simulink model "PMSM_Ld"  (R2024a)
settings: Solver=FixedStepAuto  StartTime=0.0  StopTime=0.5  FixedStep=1E-6  RelTol=1e-3
model workspace (MAT data in the model file):
  PWM_Frequency = Simulink.Parameter
  PWM_Frequency.Value = 30000
  PWM_Frequency.Complexity = 'real'
  PWM_Frequency.Dimensions = [1 1]
  PWM_Frequency.DataType = 'double'
  TimerPeriod = 0.1
values from neighbouring files (symbols this model uses):
  Flux = 0.01837    [Flux_Nonsensor_data_new.m]
undefined symbols (not defined in the file or in its folder): Down, Up
libraries: eePwmGenerator x4, spsDCVoltageSourceLib x1, spsPermanentMagnetSynchronousMachineLib x1, spsUniversalBridgeLib x1, sps_lib x1, eeGeneralControl x1
settings Model: Creator=shish  LastModifiedBy=shish

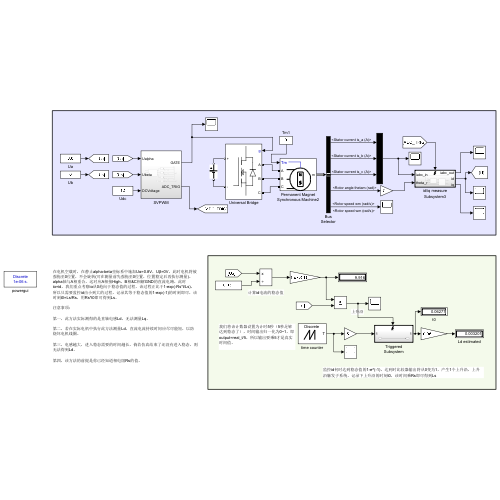
[thumbnail: Simulink's stored preview of the top-level diagram]
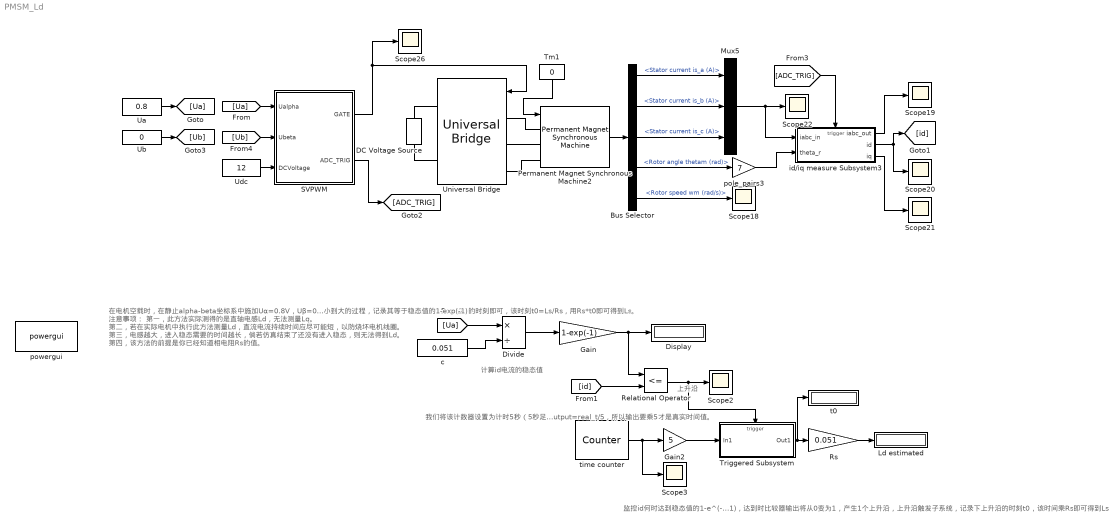
== system PMSM_Ld ==
  note: 我们将该计数器设置为计时5秒（5秒足够达到稳态了），时间输出归一化为0~1，即output=real_t/5，所以输出要乘5才是真实时间值。
  note: 上升沿
  note: 监控id何时达到稳态值的1-e^(-1)，达到时比较器输出将从0变为1，产生1个上升沿，上升沿触发子系统，记录下上升沿的时刻t0，该时间乘Rs即可得到Ls
  note: 计算id电流的稳态值
  note: 在电机空载时，在静止alpha-beta坐标系中施加Uα=0.8V，Uβ=0V，此时电机将被强拖至0位置，不会旋转(可在测量前先强拖至0位置，位置稳定后再执行测量)。alpha轴与A相重合，这对应A相接High，B相&C相解GND的直流电路，此时iα=id，我们重点考察iα从0趋向于稳态值的过程，该过程正比于1-exp(-Rs*t/Ls)，所以只需要监控id由小到大的过程，记录其等于稳态值的1-exp(-1)的时刻即可，该时刻t0=Ls/Rs，用Rs*t0即可得到Ls。
      |
      | 注意事项：
      |
      | 第一，此方法实际测得的是直轴电感Ld，无法测量Lq。
      |
      | 第二，若在实际电机中执行此方法测量Ld，直流电流持续时间应尽可能短，以防烧坏电机线圈。
      |
      | 第三，电感越大，进入稳态需要的时间越长，倘若仿真结束了还没有进入稳态，则无法得到Ld。
      |
      | 第四，该方法的前提是你已经知道相电阻Rs的值。
  " c" : Constant  Value=0.051
  Bus Selector : BusSelector  OutputSignals=Stator current is_a (A),Stator current is_b (A),Stator current is_c (A),Rotor angle thetam (rad),Rotor speed wm (rad/s)
  DC Voltage Source : spsDCVoltageSourceLib/DC Voltage Source  Amplitude=12  Measurements=Voltage
  Display : Display
  Divide : Product  Inputs=*/
  Gain : Gain  Gain=1-exp(-1)
  Gain2 : Gain  Gain=5
  Ld estimated : Display
  Mux5 : Mux  Inputs=3
  Permanent Magnet Synchronous Machine2 : spsPermanentMagnetSynchronousMachineLib/Permanent Magnet Synchronous Machine  NbPhases=3  FluxDistribution=Sinusoidal  RotorType=Salient-pole  MechanicalLoad=Torque Tm  PresetModel=No  ShowDetailedParameters=on  MeasurementBus=off  Resistance=0.05  Inductance=8.5e-3  dqInductances=[3.2e-3,1.8e-3]  La=0.000395  MachineConstant=Flux linkage established by magnets (V.s)  Flux=0.00012  VoltageCst=0.15236  TorqueCst=0.00126  Flat=120  Mechanical=[0.000012 0.000005 7 0]  PolePairs=4  InitialConditions=[0,0,0,0]  InitialConditions5ph=[0 0 0 0 0 0]  RefAngle=Aligned with phase A axis (original Park)  IterativeDiscreteModel=Trapezoidal non iterative  TsBlock=-1  TsPowergui=0
  Relational Operator : RelationalOperator  Operator=<=  OutDataTypeStr=boolean  RndMeth=Simplest  InputSameDT=off
  Rs : Gain  Gain=0.051
  SVPWM : Subsystem
  Scope{2..3,18..22,26} (8 alike) : Scope
  Tm1 : Constant  Value=0
  Triggered Subsystem : Subsystem  TreatAsAtomicUnit=on
  Ua : Constant  Value=0.8
  Ub : Constant  Value=0
  Udc : Constant  Value=12
  Universal Bridge : spsUniversalBridgeLib/Universal Bridge  Arms=3  SnubberResistance=1e5  SnubberCapacitance=inf  Device=MOSFET / Diodes  Ron=1e-3  Lon=0  ForwardVoltages="[  0  0  ]"  ForwardVoltage=0  GTOparameters=[ 10e-6 , 20e-6 ]  IGBTparameters=[ 1e-6 , 2e-6 ]  Measurements=None  Measurements_2=None  converterType=Rectifier
  id/iq measure Subsystem3 : Subsystem  TreatAsAtomicUnit=on
  pole_pairs3 : Gain  Gain=7
  powergui : sps_lib/powergui  Priority=1  SimulationMode=Discrete  SampleTime=1e-6  frequency=60  Iterations=50  frequencyindice=0  Pbase=100e6  ErrMax=1e-4  UnitsV=kV  UnitsW=MW  buscounter=0  FunctionMessages=off  echomessages=off  EnableUseOfTLC=off  CurrentSourceSwitches=off  DisableSnubberDevices=off  DisableRonSwitches=off  DisableVfSwitches=off  DisplayEquations=off  AutomaticDiscreteSolvers=off  SolverType=Tustin/Backward Euler (TBE)  Interpol=off  ExternalGateDelay=off  methode=off  Ts=100  x0status=blocks  SPID=on  SwTol=0  HookPort=off  NonlinearTolerance=1e-4  nMaxIteration=100  ContinueOnMaxIteration=off  RestoreLinks=warning  ResistiveCurrentMeasurement=off  Frange=[0:2:500]  Ylog=off  Xlog=on  ShowGrid=off  save=off  variable=ZData  structure=0  ZoomFFT=off  StartTime=0.0  cycles=1  DisplayStyle=1  fundamental=60  FreqAxis=off  MaxFrequency=1000  frequencyindicesteady=1  RmsSteady=1  display=off
  t0 : Display
  time counter : eeGeneralControl/Counter  CarrCount=Up  Range=[0 1]  Tper=5  Tdelay=0  Ts=0.000001
      settings: LibrarySourceBlock=ee_sl_lib/General Control/Counter
  wires:
  Bus Selector/5 -> Scope18/1  "<Rotor speed wm (rad/s)>"
  Bus Selector/3 -> Mux5/3  "<Stator current is_c (A)>"
  Permanent Magnet Synchronous Machine2/1 -> Bus Selector/1
  Bus Selector/4 -> pole_pairs3/1  "<Rotor angle thetam (rad)>"
  Udc/1 -> SVPWM/3(DCVoltage)
  id/iq measure Subsystem3/1(iabc_out) -> Scope19/1
  Bus Selector/2 -> Mux5/2  "<Stator current is_b (A)>"
  Mux5/1 -> Scope22/1, id/iq measure Subsystem3/1(iabc_in)
  SVPWM/1(GATE) -> Universal Bridge/1, Scope26/1
  Bus Selector/1 -> Mux5/1  "<Stator current is_a (A)>"
  pole_pairs3/1 -> id/iq measure Subsystem3/2(theta_r)
  id/iq measure Subsystem3/2(id) -> [id], Scope20/1
  id/iq measure Subsystem3/3(iq) -> Scope21/1
  [Ua] -> SVPWM/1(Ualpha)
  [Ua] -> Divide/1
  " c"/1 -> Divide/2
  Divide/1 -> Gain/1
  Gain/1 -> Relational Operator/1, Display/1
  SVPWM/2(ADC_TRIG) -> [ADC_TRIG]
  [ADC_TRIG] -> id/iq measure Subsystem3/Trigger
  [id] -> Relational Operator/2
  Relational Operator/1 -> Triggered Subsystem/Trigger, Scope2/1
  time counter/1 -> Gain2/1, Scope3/1
  Triggered Subsystem/1(Out1) -> t0/1, Rs/1
  Rs/1 -> Ld estimated/1
  Ua/1 -> [Ua]
  Gain2/1 -> Triggered Subsystem/1(In1)
  [Ub] -> SVPWM/2(Ubeta)
  Ub/1 -> [Ub]
  Tm1/1 -> Permanent Magnet Synchronous Machine2/1
  connections:
  Universal Bridge/LConn2 -- Permanent Magnet Synchronous Machine2/LConn2
  Universal Bridge/LConn1 -- Permanent Magnet Synchronous Machine2/LConn1
  Universal Bridge/LConn3 -- Permanent Magnet Synchronous Machine2/LConn3
  DC Voltage Source/LConn1 -- Universal Bridge/RConn2
  DC Voltage Source/RConn1 -- Universal Bridge/RConn1

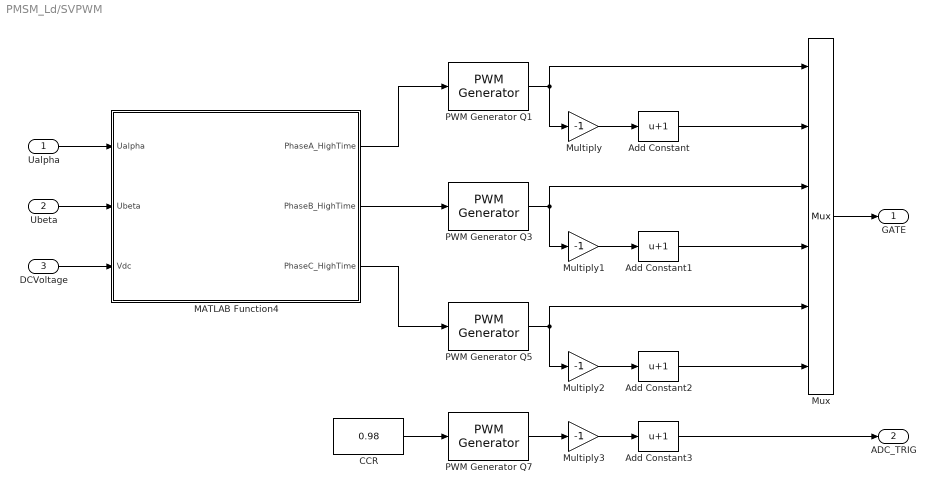
== system PMSM_Ld/SVPWM ==
  Ualpha : Inport
  Ubeta : Inport  Port=2
  DCVoltage : Inport  Port=3
  Add Constant{,1..3} (4 alike) : Bias  Bias=1  SaturateOnIntegerOverflow=off
  CCR : Constant  Value=0.98
  MATLAB Function4 : MATLAB Function  TreatAsAtomicUnit=on
  Multiply{,1..3} (4 alike) : Gain  Gain=-1
  Mux : Mux  Inputs=6
  PWM Generator Q{1,3,5,7} (4 alike) : eePwmGenerator/PWM Generator  CarrCount=Up-Down  Tper=1.0/PWM_Frequency  Tdelay=0  Ts=1E-6
  GATE : Outport
  ADC_TRIG : Outport  Port=2
  wires:
  PWM Generator Q5/1 -> Mux/5, Multiply2/1
  PWM Generator Q1/1 -> Multiply/1, Mux/1
  Add Constant1/1 -> Mux/4
  Ubeta/1 -> MATLAB Function4/2(Ubeta)
  DCVoltage/1 -> MATLAB Function4/3(Vdc)
  MATLAB Function4/3(PhaseC_HighTime) -> PWM Generator Q5/1
  Multiply/1 -> Add Constant/1
  Multiply2/1 -> Add Constant2/1
  Add Constant/1 -> Mux/2
  MATLAB Function4/2(PhaseB_HighTime) -> PWM Generator Q3/1
  Add Constant2/1 -> Mux/6
  Multiply1/1 -> Add Constant1/1
  MATLAB Function4/1(PhaseA_HighTime) -> PWM Generator Q1/1
  Ualpha/1 -> MATLAB Function4/1(Ualpha)
  PWM Generator Q3/1 -> Mux/3, Multiply1/1
  PWM Generator Q7/1 -> Multiply3/1
  CCR/1 -> PWM Generator Q7/1
  Add Constant3/1 -> ADC_TRIG/1
  Multiply3/1 -> Add Constant3/1
  Mux/1 -> GATE/1

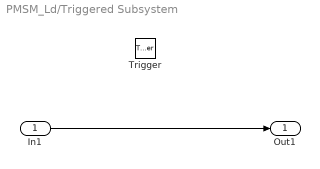
== system PMSM_Ld/Triggered Subsystem ==
  In1 : Inport
  Trigger : TriggerPort  VariantControl=(inherit)
  Out1 : Outport
  wires:
  In1/1 -> Out1/1

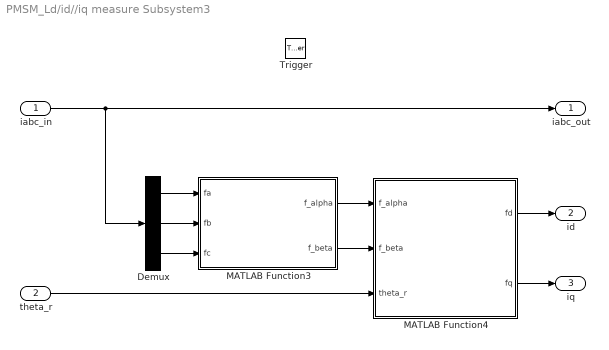
== system PMSM_Ld/id//iq measure Subsystem3 ==
  iabc_in : Inport
  theta_r : Inport  Port=2
  Trigger : TriggerPort  VariantControl=(inherit)
  Demux : Demux  Outputs=3
  MATLAB Function3 : MATLAB Function  TreatAsAtomicUnit=on
  MATLAB Function4 : MATLAB Function  TreatAsAtomicUnit=on
  iabc_out : Outport
  id : Outport  Port=2
  iq : Outport  Port=3
  wires:
  iabc_in/1 -> Demux/1, iabc_out/1
  Demux/3 -> MATLAB Function3/3(fc)
  Demux/2 -> MATLAB Function3/2(fb)
  Demux/1 -> MATLAB Function3/1(fa)
  MATLAB Function3/1(f_alpha) -> MATLAB Function4/1(f_alpha)
  MATLAB Function3/2(f_beta) -> MATLAB Function4/2(f_beta)
  theta_r/1 -> MATLAB Function4/3(theta_r)
  MATLAB Function4/1(fd) -> id/1
  MATLAB Function4/2(fq) -> iq/1

== matlab function PMSM_Ld/SVPWM/MATLAB Function4 ==
  data: Ualpha input; PhaseA_HighTime output; Ubeta input; Vdc input; PhaseB_HighTime output; PhaseC_HighTime output
function [PhaseA_HighTime,PhaseB_HighTime,PhaseC_HighTime] = SVPWM_calculate(Ualpha,Ubeta,Vdc)

% unit:V %

%step 1,which sector?%
if Ualpha >= 0
    %sector=1,2,5,6%
    if Ubeta >= 0
        %sector=1,2%
        if Ubeta > sqrt(3)*Ualpha
            sector=2;
        else
            sector=1;
        end
    else
        %sector=5,6%
        if -Ubeta > sqrt(3)*Ualpha
            sector=5;
        else
            sector=6;
        end
    end
else
    %sector=2,3,4,5%
    if Ubeta >= 0
        %sector=2,3%
        if Ubeta > -sqrt(3)*Ualpha
            sector=2;
        else
            sector=3;
        end
    else
        %sector=4,5%
        if -Ubeta > -sqrt(3)*Ualpha
            sector=5;
        else
            sector=4;
        end
    end
end

%step 2,vector decompose%
v1 = (2*Vdc/3)*[ 1,0];
v2 = (2*Vdc/3)*[ 0.5, 0.5*sqrt(3)];
v3 = (2*Vdc/3)*[-0.5, 0.5*sqrt(3)];
v4 = (2*Vdc/3)*[-1,0];
v5 = (2*Vdc/3)*[-0.5,-0.5*sqrt(3)];
v6 = (2*Vdc/3)*[ 0.5,-0.5*sqrt(3)];

if sector == 1
    vm=v1;vn=v2;
elseif sector == 2
    vm=v2;vn=v3;
elseif sector == 3
    vm=v3;vn=v4;
elseif sector == 4
    vm=v4;vn=v5;
elseif sector == 5
    vm=v5;vn=v6;
else
    vm=v6;vn=v1;
end

cm = (Ualpha*vn(2) - Ubeta*vn(1))/(vm(1)*vn(2) - vm(2)*vn(1));

if abs(vn(1))>1e-7
    cn = (Ualpha-cm*vm(1))/vn(1);
else
    cn = (Ubeta-cm*vm(2))/vn(2);
end
c_summ = cm+cn;
% if c_summ > 1
%     cm = cm/c_summ;
%     cn = cn/c_summ;
% end
if c_summ > 0.95
    cm = 0.95*cm/c_summ;
    cn = 0.95*cn/c_summ;
end

c0 = (1-cm-cn);
c0 = 0.5*c0;
c7 = c0;

%step 3,duty cycle%
if sector == 1
    %v1:100  v2:110%
    PhaseA_HighTime = cm+cn+c7;
    PhaseB_HighTime = cn+c7;
    PhaseC_HighTime = c7;
elseif sector == 2
    %v2:110  v3:010%
    PhaseA_HighTime = cm+c7;
    PhaseB_HighTime = cm+cn+c7;
    PhaseC_HighTime = c7;
elseif sector == 3
    %v3:010  v4:011%
    PhaseA_HighTime = c7;
    PhaseB_HighTime = cm+cn+c7;
    PhaseC_HighTime = cn+c7;
elseif sector == 4
    %v4:011  v5:001%
    PhaseA_HighTime = c7;
    PhaseB_HighTime = cm+c7;
    PhaseC_HighTime = cm+cn+c7;
elseif sector == 5
    %v5:001  v6:101%
    PhaseA_HighTime = cn+c7;
    PhaseB_HighTime = c7;
    PhaseC_HighTime = cm+cn+c7;
else
    %v6:101  v1:100%
    PhaseA_HighTime = cm+cn+c7;
    PhaseB_HighTime = c7;
    PhaseC_HighTime = cm+c7;
end

== matlab function PMSM_Ld/id//iq measure Subsystem3/MATLAB Function3 ==
  data: fa input; f_alpha output; fb input; fc input; f_beta output
function [f_alpha,f_beta]= ABC_to_AlphaBeta(fa,fb,fc)
f_alpha = (2/3)*(fa-0.5*(fb+fc));
f_beta = (2/3)*(0.5*sqrt(3)*(fb-fc));

== matlab function PMSM_Ld/id//iq measure Subsystem3/MATLAB Function4 ==
  data: f_alpha input; fd output; f_beta input; fq output; theta_r input
function [fd,fq]= AlphaBeta_to_dq(f_alpha,f_beta,theta_r)

c = cos(theta_r);
s = sin(theta_r);
fd =  c*f_alpha + s*f_beta;
fq = -s*f_alpha + c*f_beta;
